simulink library "lib_StateEstimation"  (R2017b)
settings: Solver=VariableStepAuto  StartTime=0.0  StopTime=10.0  RelTol=1e-3
undefined symbols (not defined in the file): accel_true_bias_init, accel_true_bias_noise_std, accel_true_noise_std, cassieParameters, gyro_true_bias_init, gyro_true_bias_noise_std, gyro_true_noise_std, RIEKF_InitFcn
libraries: simulink x6
settings Model: Creator=Ross Hartley  LastModifiedBy=Ross Hartley
settings CodeAppCC: StateflowObjectComments=on

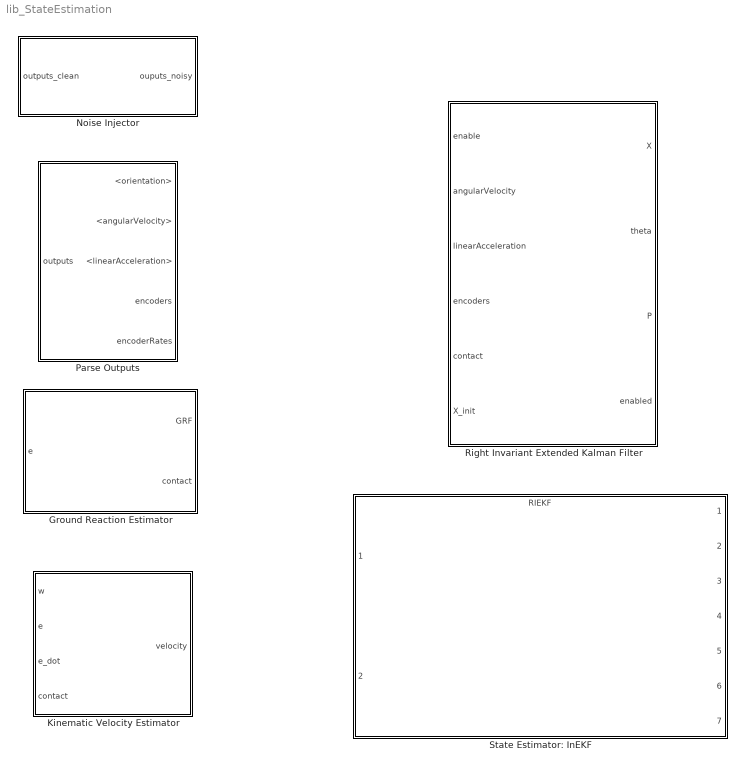
== system lib_StateEstimation ==
  Ground Reaction Estimator : Subsystem
  Kinematic Velocity Estimator : Subsystem
  Noise Injector : Subsystem
  Parse Outputs : Subsystem
  Right Invariant Extended Kalman Filter : Subsystem  InitFcn=RIEKF_InitFcn;
  State Estimator: InEKF : ModelReference  ModelNameDialog=RIEKF.slx  SimulationMode=Normal  ModelReferenceVersion=1.1533
      mask Display:
      | image('BaseContactFrames.png');
      | port_label('input',1,'enable');
      | port_label('input',2,'outputs');
      | port_label('output',1,'q');
      | port_label('output',2,'dq');
      | port_label('output',3,'GRF');
      | port_label('output',4,'X');
      | port_label('output',5,'theta');
      | port_label('output',6,'P');
      | port_label('output',7,'enabled');

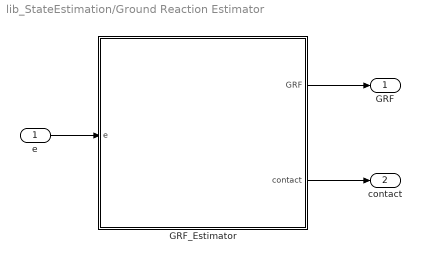
== system lib_StateEstimation/Ground Reaction Estimator ==
  e : Inport
  GRF_Estimator : MATLAB Function  TreatAsAtomicUnit=on
  GRF : Outport
  contact : Outport  Port=2
  wires:
  GRF_Estimator/1(GRF) -> GRF/1
  GRF_Estimator/2(contact) -> contact/1
  e/1 -> GRF_Estimator/1(e)

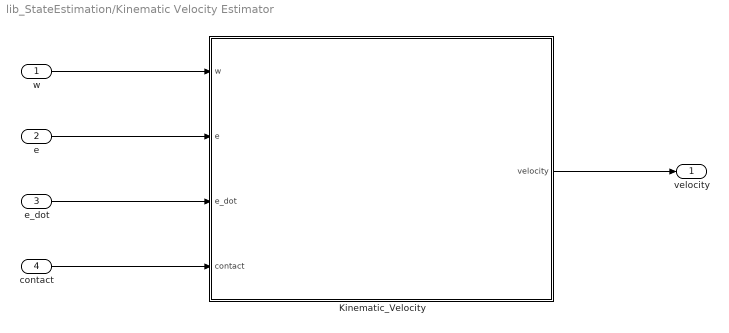
== system lib_StateEstimation/Kinematic Velocity Estimator ==
  w : Inport
  e : Inport  Port=2
  e_dot : Inport  Port=3
  contact : Inport  Port=4
  Kinematic_Velocity : MATLAB Function  TreatAsAtomicUnit=on
  velocity : Outport
  wires:
  e/1 -> Kinematic_Velocity/2(e)
  e_dot/1 -> Kinematic_Velocity/3(e_dot)
  Kinematic_Velocity/1(velocity) -> velocity/1
  contact/1 -> Kinematic_Velocity/4(contact)
  w/1 -> Kinematic_Velocity/1(w)

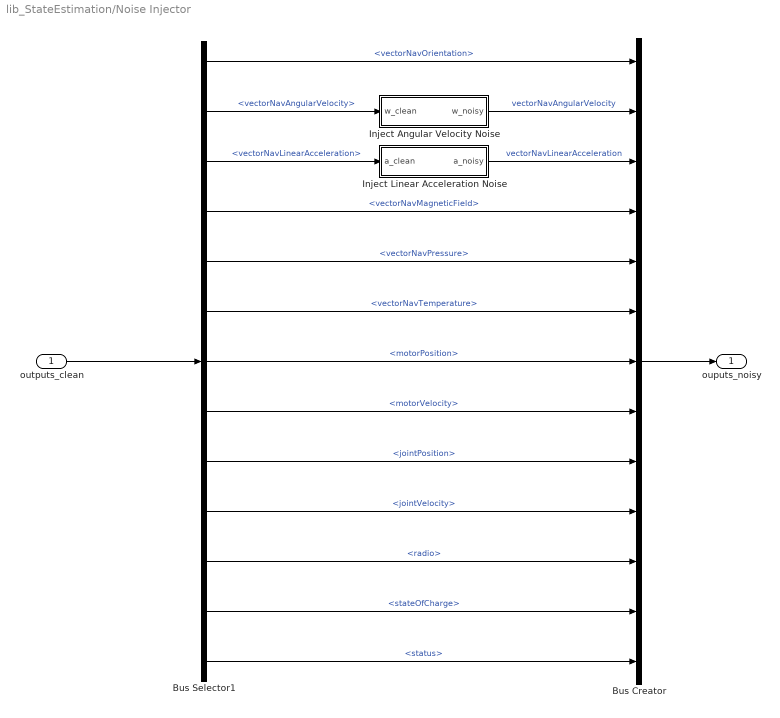
== system lib_StateEstimation/Noise Injector ==
  outputs_clean : Inport
  Bus Creator : BusCreator  Inputs=13  OutDataTypeStr=Bus: cassieOutputsBus
  Bus Selector1 : BusSelector  OutputSignals=vectorNavOrientation,vectorNavAngularVelocity,vectorNavLinearAcceleration,vectorNavMagneticField,vectorNavPressure,vectorNavTemperature,motorPosition,motorVelocity,jointPosition,jointVelocity,radio,stateOfCharge,status
  Inject Angular Velocity Noise : Subsystem
  Inject Linear Acceleration Noise : Subsystem
  ouputs_noisy : Outport
  wires:
  Inject Linear Acceleration Noise/1(a_noisy) -> Bus Creator/3  "vectorNavLinearAcceleration"
  Inject Angular Velocity Noise/1(w_noisy) -> Bus Creator/2  "vectorNavAngularVelocity"
  Bus Selector1/2 -> Inject Angular Velocity Noise/1(w_clean)  "<vectorNavAngularVelocity>"
  Bus Creator/1 -> ouputs_noisy/1
  Bus Selector1/11 -> Bus Creator/11  "<radio>"
  Bus Selector1/12 -> Bus Creator/12  "<stateOfCharge>"
  Bus Selector1/9 -> Bus Creator/9  "<jointPosition>"
  Bus Selector1/13 -> Bus Creator/13  "<status>"
  Bus Selector1/10 -> Bus Creator/10  "<jointVelocity>"
  Bus Selector1/8 -> Bus Creator/8  "<motorVelocity>"
  Bus Selector1/3 -> Inject Linear Acceleration Noise/1(a_clean)  "<vectorNavLinearAcceleration>"
  Bus Selector1/4 -> Bus Creator/4  "<vectorNavMagneticField>"
  Bus Selector1/7 -> Bus Creator/7  "<motorPosition>"
  Bus Selector1/5 -> Bus Creator/5  "<vectorNavPressure>"
  Bus Selector1/6 -> Bus Creator/6  "<vectorNavTemperature>"
  Bus Selector1/1 -> Bus Creator/1  "<vectorNavOrientation>"
  outputs_clean/1 -> Bus Selector1/1

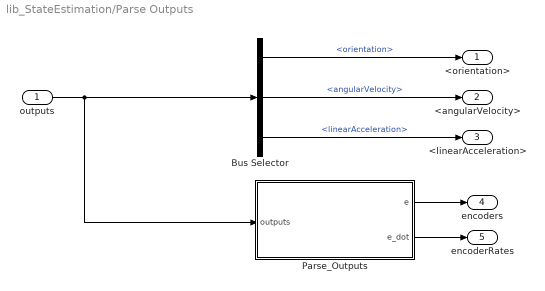
== system lib_StateEstimation/Parse Outputs ==
  outputs : Inport
  Bus Selector : BusSelector  OutputSignals=pelvis.vectorNav.orientation,pelvis.vectorNav.angularVelocity,pelvis.vectorNav.linearAcceleration
  Parse_Outputs : MATLAB Function  TreatAsAtomicUnit=on
  <orientation> : Outport
  <angularVelocity> : Outport  Port=2
  <linearAcceleration> : Outport  Port=3
  encoders : Outport  Port=4
  encoderRates : Outport  Port=5
  wires:
  outputs/1 -> Parse_Outputs/1(outputs), Bus Selector/1
  Parse_Outputs/2(e_dot) -> encoderRates/1
  Parse_Outputs/1(e) -> encoders/1
  Bus Selector/2 -> <angularVelocity>/1  "<angularVelocity>"
  Bus Selector/3 -> <linearAcceleration>/1  "<linearAcceleration>"
  Bus Selector/1 -> <orientation>/1  "<orientation>"

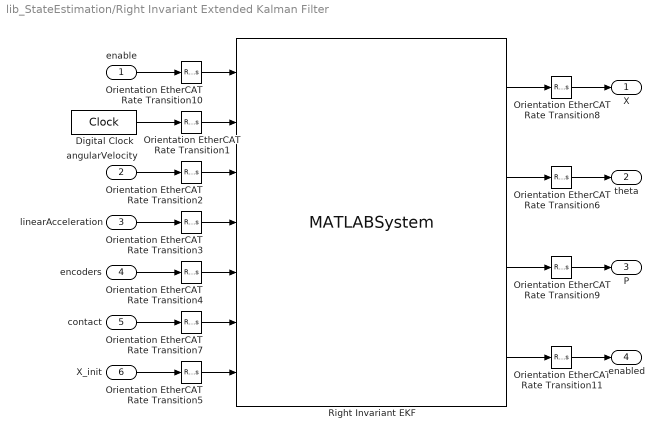
== system lib_StateEstimation/Right Invariant Extended Kalman Filter ==
  enable : Inport
  angularVelocity : Inport  Port=2
  linearAcceleration : Inport  Port=3
  encoders : Inport  Port=4
  contact : Inport  Port=5
  X_init : Inport  Port=6
  Digital Clock : DigitalClock  SampleTime=-1
  Orientation EtherCAT Rate Transition{1..5,7,10} (7 alike) : RateTransition  Deterministic=off  OutPortSampleTime=EKF_SampleTime
  Orientation EtherCAT Rate Transition{6,8..9,11} (4 alike) : RateTransition  Deterministic=off  OutPortSampleTime=0.0005
  Right Invariant EKF : MATLABSystem  System=RightInvariantEKF  static_bias_initialization=static_bias_initialization  ekf_update_enabled=ekf_update_enabled  enable_bias_estimation=enable_bias_estimation  gyro_noise_std=gyro_noise_std  gyro_bias_noise_std=gyro_bias_noise_std  accel_noise_std=accel_noise_std  accel_bias_noise_std=accel_bias_noise_std  contact_noise_std=contact_noise_std  encoder_noise_std=encoder_noise_std  gyro_bias_init=gyro_bias_init  accel_bias_init=accel_bias_init  prior_base_pose_std=prior_base_pose_std  prior_base_velocity_std=prior_base_velocity_std  prior_contact_position_std=prior_contact_position_std  prior_gyro_bias_std=prior_gyro_bias_std  prior_accel_bias_std=prior_accel_bias_std  prior_forward_kinematics_std=prior_forward_kinematics_std  SimulateUsing=Code generation
      mask Type: RightInvariantEKF
      mask Display:
      | disp('RightInvariantEKF');
      | port_label('input',1,'enable');
      | port_label('input',2,'t');
      | port_label('input',3,'w');
      | port_label('input',4,'a');
      | port_label('input',5,'encoders');
      | port_label('input',6,'contact');
      | port_label('input',7,'X_init');
      | port_label('output',1,'X');
      | port_label('output',2,'theta');
      | port_label('output',3,'P');
      | port_label('output',4,'enabled');
  X : Outport
  theta : Outport  Port=2
  P : Outport  Port=3
  enabled : Outport  Port=4
  wires:
  Orientation EtherCAT Rate Transition2/1 -> Right Invariant EKF/3
  Orientation EtherCAT Rate Transition4/1 -> Right Invariant EKF/5
  Orientation EtherCAT Rate Transition5/1 -> Right Invariant EKF/7
  Right Invariant EKF/4 -> Orientation EtherCAT Rate Transition11/1
  contact/1 -> Orientation EtherCAT Rate Transition7/1
  Orientation EtherCAT Rate Transition10/1 -> Right Invariant EKF/1
  Right Invariant EKF/3 -> Orientation EtherCAT Rate Transition9/1
  Orientation EtherCAT Rate Transition11/1 -> enabled/1
  Orientation EtherCAT Rate Transition7/1 -> Right Invariant EKF/6
  Right Invariant EKF/2 -> Orientation EtherCAT Rate Transition6/1
  Orientation EtherCAT Rate Transition1/1 -> Right Invariant EKF/2
  Right Invariant EKF/1 -> Orientation EtherCAT Rate Transition8/1
  Orientation EtherCAT Rate Transition3/1 -> Right Invariant EKF/4
  Orientation EtherCAT Rate Transition6/1 -> theta/1
  encoders/1 -> Orientation EtherCAT Rate Transition4/1
  linearAcceleration/1 -> Orientation EtherCAT Rate Transition3/1
  Orientation EtherCAT Rate Transition9/1 -> P/1
  angularVelocity/1 -> Orientation EtherCAT Rate Transition2/1
  Orientation EtherCAT Rate Transition8/1 -> X/1
  Digital Clock/1 -> Orientation EtherCAT Rate Transition1/1
  enable/1 -> Orientation EtherCAT Rate Transition10/1
  X_init/1 -> Orientation EtherCAT Rate Transition5/1

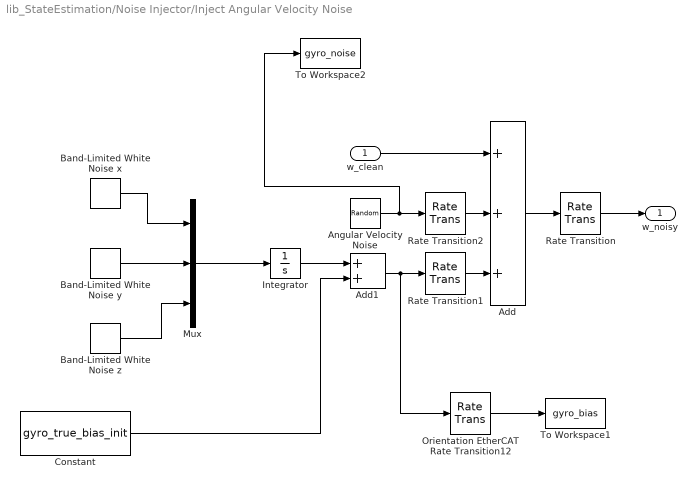
== system lib_StateEstimation/Noise Injector/Inject Angular Velocity Noise ==
  w_clean : Inport
  Add : Sum  Inputs=+++
  Add1 : Sum
  Angular Velocity Noise : RandomNumber  Mean=[0;0;0]  Variance=[gyro_true_noise_std(1)^2; gyro_true_noise_std(2)^2; gyro_true_noise_std(3)^2]  Seed=[7;8;9]  SampleTime=cassieParameters.vectorNavSampleTime
  Band-Limited White Noise x : simulink/Sources/Band-Limited White Noise  Cov=[gyro_true_bias_noise_std(1)^2]  Ts=cassieParameters.etherCatSampleTime  seed=[1]
  Band-Limited White Noise y : simulink/Sources/Band-Limited White Noise  Cov=[gyro_true_bias_noise_std(2)^2]  Ts=cassieParameters.etherCatSampleTime  seed=[2]
  Band-Limited White Noise z : simulink/Sources/Band-Limited White Noise  Cov=[gyro_true_bias_noise_std(3)^2]  Ts=cassieParameters.etherCatSampleTime  seed=[3]
  Constant : Constant  Value=gyro_true_bias_init
  Integrator : Integrator  InitialCondition=[0;0;0]
  Mux : Mux  Inputs=3
  Orientation EtherCAT Rate Transition12 : RateTransition  Deterministic=off  OutPortSampleTime=CassieParameters.etherCatSampleTime
  Rate Transition : RateTransition  OutPortSampleTime=cassieParameters.etherCatSampleTime
  Rate Transition1 : RateTransition  Deterministic=off  OutPortSampleTime=cassieParameters.etherCatSampleTime
  Rate Transition2 : RateTransition  Deterministic=off  OutPortSampleTime=cassieParameters.etherCatSampleTime
  To Workspace1 : ToWorkspace  VariableName=gyro_bias  SaveFormat=Timeseries  SampleTime=-1
  To Workspace2 : ToWorkspace  VariableName=gyro_noise  SaveFormat=Structure With Time  SampleTime=-1
  w_noisy : Outport
  wires:
  Add/1 -> Rate Transition/1
  Rate Transition/1 -> w_noisy/1
  Mux/1 -> Integrator/1
  Band-Limited White Noise z/1 -> Mux/3
  Band-Limited White Noise y/1 -> Mux/2
  Band-Limited White Noise x/1 -> Mux/1
  Integrator/1 -> Add1/1
  Angular Velocity Noise/1 -> To Workspace2/1, Rate Transition2/1
  w_clean/1 -> Add/1
  Add1/1 -> Orientation EtherCAT Rate Transition12/1, Rate Transition1/1
  Constant/1 -> Add1/2
  Rate Transition1/1 -> Add/3
  Rate Transition2/1 -> Add/2
  Orientation EtherCAT Rate Transition12/1 -> To Workspace1/1

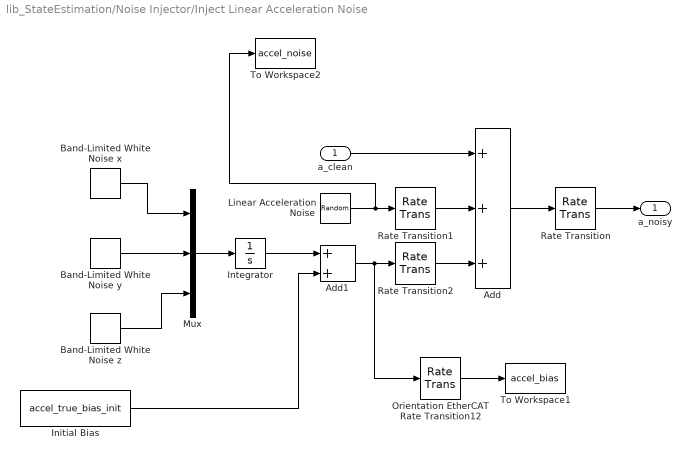
== system lib_StateEstimation/Noise Injector/Inject Linear Acceleration Noise ==
  a_clean : Inport
  Add : Sum  Inputs=+++
  Add1 : Sum
  Band-Limited White Noise x : simulink/Sources/Band-Limited White Noise  Cov=[accel_true_bias_noise_std(1)^2]  Ts=cassieParameters.etherCatSampleTime  seed=[4]
  Band-Limited White Noise y : simulink/Sources/Band-Limited White Noise  Cov=[accel_true_bias_noise_std(2)^2]  Ts=cassieParameters.etherCatSampleTime  seed=[5]
  Band-Limited White Noise z : simulink/Sources/Band-Limited White Noise  Cov=[accel_true_bias_noise_std(3)^2]  Ts=cassieParameters.etherCatSampleTime  seed=[6]
  Initial Bias : Constant  Value=accel_true_bias_init
  Integrator : Integrator  InitialCondition=[0;0;0]
  Linear Acceleration Noise : RandomNumber  Mean=[0;0;0]  Variance=[accel_true_noise_std(1)^2; accel_true_noise_std(2)^2; accel_true_noise_std(3)^2]  Seed=[10;11;12]  SampleTime=cassieParameters.vectorNavSampleTime
  Mux : Mux  Inputs=3
  Orientation EtherCAT Rate Transition12 : RateTransition  Deterministic=off  OutPortSampleTime=CassieParameters.etherCatSampleTime
  Rate Transition : RateTransition  OutPortSampleTime=cassieParameters.etherCatSampleTime
  Rate Transition1 : RateTransition  Deterministic=off  OutPortSampleTime=cassieParameters.etherCatSampleTime
  Rate Transition2 : RateTransition  Deterministic=off  OutPortSampleTime=cassieParameters.etherCatSampleTime
  To Workspace1 : ToWorkspace  VariableName=accel_bias  SaveFormat=Timeseries  SampleTime=-1
  To Workspace2 : ToWorkspace  VariableName=accel_noise  SaveFormat=Structure With Time  SampleTime=-1
  a_noisy : Outport
  wires:
  Add/1 -> Rate Transition/1
  Integrator/1 -> Add1/1
  Mux/1 -> Integrator/1
  Band-Limited White Noise z/1 -> Mux/3
  Band-Limited White Noise y/1 -> Mux/2
  Band-Limited White Noise x/1 -> Mux/1
  Linear Acceleration Noise/1 -> To Workspace2/1, Rate Transition1/1
  a_clean/1 -> Add/1
  Initial Bias/1 -> Add1/2
  Add1/1 -> Orientation EtherCAT Rate Transition12/1, Rate Transition2/1
  Rate Transition1/1 -> Add/2
  Rate Transition2/1 -> Add/3
  Orientation EtherCAT Rate Transition12/1 -> To Workspace1/1
  Rate Transition/1 -> a_noisy/1

== matlab function lib_StateEstimation/Kinematic Velocity Estimator/Kinematic_Velocity ==
  data: w input; e input; e_dot input; contact input; velocity output
function velocity  = Kinematic_Velocity(w, e, e_dot, contact)
% Kinematic Velocity Estimator

if contact(1) == 1
    pL = p_VectorNav_to_LeftToeBottom(e); % {I}_p_{IL}
    J_pL = J_VectorNav_to_LeftToeBottom(e);
    velocity = -J_pL(1:3,:)*e_dot - Angles.skew(w)*pL(1:3,:); % {I}_v_{WI}
elseif contact(2) == 1
    pR = p_VectorNav_to_RightToeBottom(e); % {I}_p_{IR}
    J_pR = J_VectorNav_to_RightToeBottom(e);
    velocity = -J_pR(1:3,:)*e_dot - Angles.skew(w)*pR(1:3,:); % {I}_v_{WI}
else
    velocity = zeros(3,1);
end

end

== matlab function lib_StateEstimation/Parse Outputs/Parse_Outputs ==
  data: e output; outputs input; e_dot output
function [e, e_dot] = Extract_Encoders(outputs)   
%   Author: Ross Hartley 
%   Date:   7/03/2017
%
% Get positions
qa = CassieModule.getDriveProperty(outputs, 'position');
qj = CassieModule.getJointProperty(outputs, 'position');

% Get velocities
dqa = CassieModule.getDriveProperty(outputs, 'velocity');
dqj = CassieModule.getJointProperty(outputs, 'velocity');

% Construct State Vector
e = [qa(1:3); qa(4); qj(1); qj(2); qa(5); qa(6:8); qa(9); qj(4); qj(5); qa(10)];
e_dot = [dqa(1:3); dqa(4); dqj(1); dqj(2); dqa(5); dqa(6:8); dqa(9); dqj(4); dqj(5); dqa(10)];

end

== matlab function lib_StateEstimation/Ground Reaction Estimator/GRF_Estimator ==
  data: e input; GRF output; contact output
function [GRF, contact] = GRF_Estimator(e)
% Estimates the ground reaction force in the body frame of the robot
%
% Fe_i = (S_i * J_i^T)^{-1} * S_i * \tau_d
% 

J_pR = J_VectorNav_to_RightToeBottom(e);
J_pL = J_VectorNav_to_LeftToeBottom(e);

qs_knee_L = e(5);
qs_tarsus_L = e(4) + e(5) + e(6) - deg2rad(13);
 
qs_knee_R = e(12);
qs_tarsus_R = e(11) + e(12) + e(13) - deg2rad(13);

tau_L = -[1500; 1250].*[qs_knee_L + qs_tarsus_L; qs_tarsus_L];
tau_R = -[1500; 1250].*[qs_knee_R + qs_tarsus_R; qs_tarsus_R];

GRF_L = -[J_pL([1,3],5), J_pL([1,3],6)] \ tau_L;
GRF_R = -[J_pR([1,3],12), J_pR([1,3],13)] \ tau_R;
GRF = [GRF_L; GRF_R];  

% Detect contact using GRF
cL = scaleFactor(GRF(2), 50, 100);
cR = scaleFactor(GRF(4), 50, 100);
contact = [cL; cR];

end

function s = scaleFactor(f, tl, tu)
	%SCALEFACTOR Compute scalar (0 to 1) representing forces in leg.
	s = (clamp(f, tl, tu) - tl)/(tu - tl);
end % scaleFactor
